simulink model "AccelerationPedalPositionSensor"  (R2025a)
settings: Solver=FixedStepDiscrete  StartTime=0.0  StopTime=10.0  FixedStep=0.005  RelTol=1e-3
settings Model: Creator=z004f2se  LastModifiedBy=z004f2se
settings DataIOCC: SaveFormat=StructureWithTime
settings OptimizationCC: DefaultParameterBehavior=Inlined  EnhancedBackFolding=on  PassReuseOutputArgsAs=Individual arguments  ZeroExternalMemoryAtStartup=off  ZeroInternalMemoryAtStartup=off  OptimizeBlockOrder=speed  DifferentSizesBufferReuse=on  OptimizationCustomize=off  EfficientTunableParamExpr=on
settings DebuggingCC: ParameterTunabilityLossMsg=error
settings SFSimCC: MATLABDynamicMemAlloc=off
settings RTWCC: SystemTargetFile=autosar.tlc  GenCodeOnly=on  TemplateMakefile=ert_default_tmf  DataTypeReplacement=CDataTypesFixedWidth  Description=AUTOSAR
settings CodeAppCC: ForceParamTrailComments=on  IgnoreCustomStorageClasses=off  OperatorAnnotations=on  SimulinkDataObjDesc=on  SFDataObjDesc=on  InsertBlockDesc=on
settings STFCustomTargetCC: SystemTargetFile=autosar.tlc  TargetLangStandard=C99 (ISO)  MultiwordLength=256.0  DynamicStringBufferSize=256.0  ParMdlRefBuildCompliant=on  CompOptLevelCompliant=on  IncludeMdlTerminateFcn=off  CombineOutputUpdateFcns=on  SuppressErrorStatus=on  ERTCustomFileBanners=on  SupportNonFinite=off  SupportComplex=off  SupportContinuousTime=off  SupportNonInlinedSFcns=off  RemoveResetFunc=on  MATLABClassNameForMDSCustomization=Simulink.SoftwareTarget.ERTCustomization  AutosarCompliant=on  GRTInterface=off  UseToolchainInfoCompliant=on  LookupTableObjectStructAxisOrder=2,1,3,4,...  LUTObjectStructOrderEvenSpacing=Size,Table,Breakpoints  AutosarCompilerAbstraction=off  AutosarMatrixIOAsArray=off  AutosarSchemaVersion=4.2  DisableAUTOSARRoutinesHostLibrary=off  AutosarMaxShortNameLength=128.0
settings ERTTargetCC: ExtModeTransport=0.0  ExtModeStaticAlloc=off  ExtModeMexFile=ext_comm  ExtModeIntrfLevel=Level1  ERTCustomFileTemplate=example_file_process.tlc  BooleanTrueId=TRUE  BooleanFalseId=FALSE  TargetLangStandard=C99 (ISO)  ConcurrentExecutionCompliant=off  IncludeMdlTerminateFcn=off  SuppressErrorStatus=on  SupportNonFinite=off  SupportComplex=off  ModelStepFunctionPrototypeControlCompliant=off  CPPClassGenCompliant=off  AutosarCompliant=on  LookupTableObjectStructAxisOrder=2,1,3,4,...  LUTObjectStructOrderEvenSpacing=Size,Table,Breakpoints

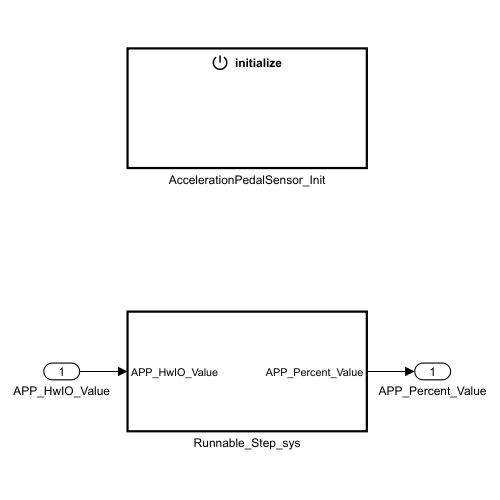
[thumbnail: Simulink's stored preview of the top-level diagram]
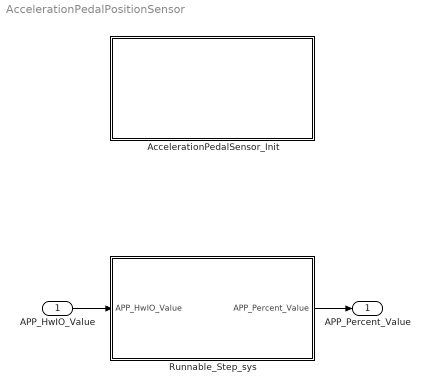
== system AccelerationPedalPositionSensor ==
  APP_HwIO_Value : Inport  OutDataTypeStr=uint16  PortDimensions=1
  AccelerationPedalSensor_Init : Subsystem
  Runnable_Step_sys : Subsystem  TreatAsAtomicUnit=on  SystemSampleTime=0.005
  APP_Percent_Value : Outport  OutDataTypeStr=single  PortDimensions=1
  wires:
  APP_HwIO_Value/1 -> Runnable_Step_sys/1(APP_HwIO_Value)
  Runnable_Step_sys/1(APP_Percent_Value) -> APP_Percent_Value/1

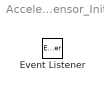
== system AccelerationPedalPositionSensor/AccelerationPedalSensor_Init ==
  Event Listener : EventListener  EventName=reset

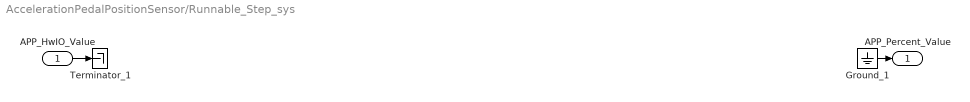
== system AccelerationPedalPositionSensor/Runnable_Step_sys ==
  APP_HwIO_Value : Inport
  Ground_1 : Ground
  Terminator_1 : Terminator
  APP_Percent_Value : Outport
  wires:
  APP_HwIO_Value/1 -> Terminator_1/1
  Ground_1/1 -> APP_Percent_Value/1
